simulink model "ball"  (R2020a)
settings: Solver=VariableStepAuto  StartTime=0.0  StopTime=10.0  RelTol=1e-3
values from neighbouring files (symbols this model uses):
  d = 0.03    [ball_and_plate_TF.m]
  g = -9.8    [ball_and_plate_TF.m]
  J = 9.99e-6    (= 9.99e-06)    [ball_and_plate_TF.m]
  L = 1.0    (= 1)    [ball_and_plate_TF.m]
  m = 0.111    [ball_and_plate_TF.m]
  R = 0.015    [ball_and_plate_TF.m]
settings Model: Creator=Allan  LastModifiedBy=Allan

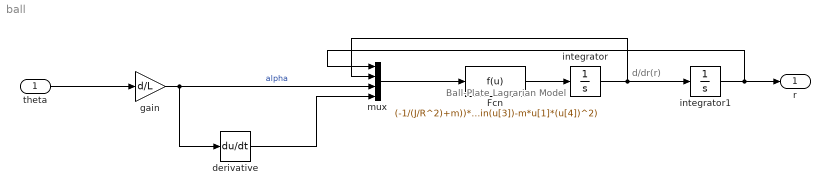
== system ball ==
  note: Ball-Plate Lagrarian Model
  note: d/dr(r)
  theta : Inport
  Fcn : Fcn  Expr=(-1/(J/R^2)+m))*(m*g*sin(u[3])-m*u[1]*(u[4])^2)
  derivative : Derivative
  gain : Gain  Gain=d/L
  integrator : Integrator
  integrator1 : Integrator
  mux : Mux
  r : Outport
  wires:
  integrator/1 -> mux/2, integrator1/1
  integrator1/1 -> mux/1, r/1
  Fcn/1 -> integrator/1
  mux/1 -> Fcn/1
  derivative/1 -> mux/4
  gain/1 -> derivative/1, mux/3  "alpha"
  theta/1 -> gain/1
